simulink model "Hood_HVAC_HIL"  (R2020b)
settings: Solver=VariableStepAuto  StartTime=0.0  StopTime=inf  RelTol=1e-3
libraries: simulink x2
settings Model: Creator=99003785  LastModifiedBy=99003785

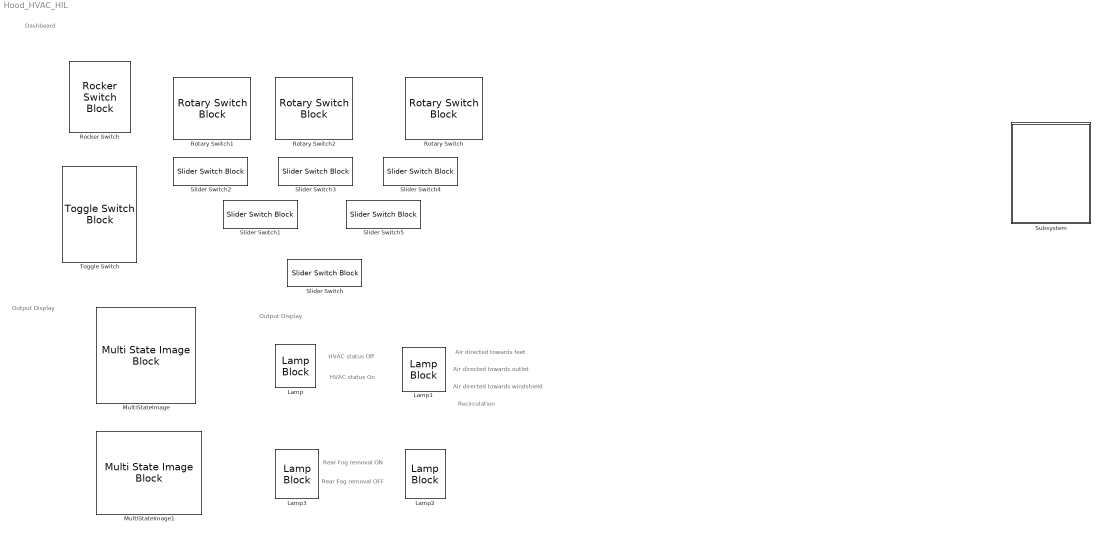
== system Hood_HVAC_HIL ==
  note: Rear Fog removal ON
  note: Air directed towards feet
  note: Air directed towards outlet
  note: HVAC status Off
  note: Output Display
  note: Recirculation
  note: Output Display
  note: Air directed towards windshield
  note: Dashboard
  note: HVAC status On
  note: Rear Fog removal OFF
  Lamp{,1..3} (4 alike) : LampBlock
  MultiStateImage : MultiStateImageBlock
  MultiStateImage1 : MultiStateImageBlock
  Rocker Switch : RockerSwitchBlock
      settings: Values={{'On', 'Off'}, [1 0]}
  Rotary Switch : RotarySwitchBlock
      settings: Values={{'Off', 'Low', 'Medium', 'High'}, [0 1 2 3]}
  Rotary Switch1 : RotarySwitchBlock
      settings: Values={{'Off', 'Low', 'Medium', 'High'}, [0 1 2 3]}
  Rotary Switch2 : RotarySwitchBlock
      settings: Values={{'Off', 'AC', 'Heater', 'Air-Vent'}, [0 1 2 3]}
  Slider Switch{,1..5} (6 alike) : SliderSwitchBlock
      settings: Values={{'Off', 'On'}, [0 1]}
  Subsystem : Subsystem
  Toggle Switch : ToggleSwitchBlock
      settings: Values={{'Off', 'On'}, [0 1]}

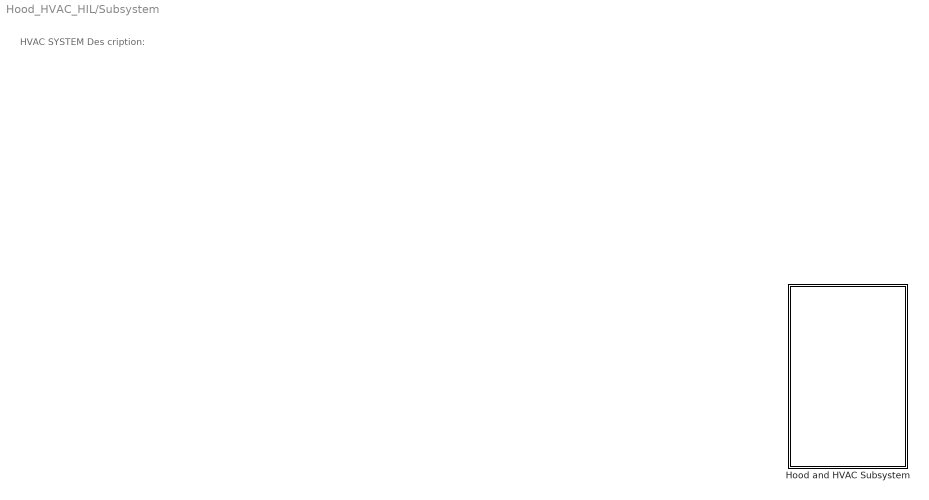
== system Hood_HVAC_HIL/Subsystem ==
  note: HVAC SYSTEM
      |
      | Des cription:
  Hood and HVAC Subsystem : Subsystem  TreatAsAtomicUnit=on

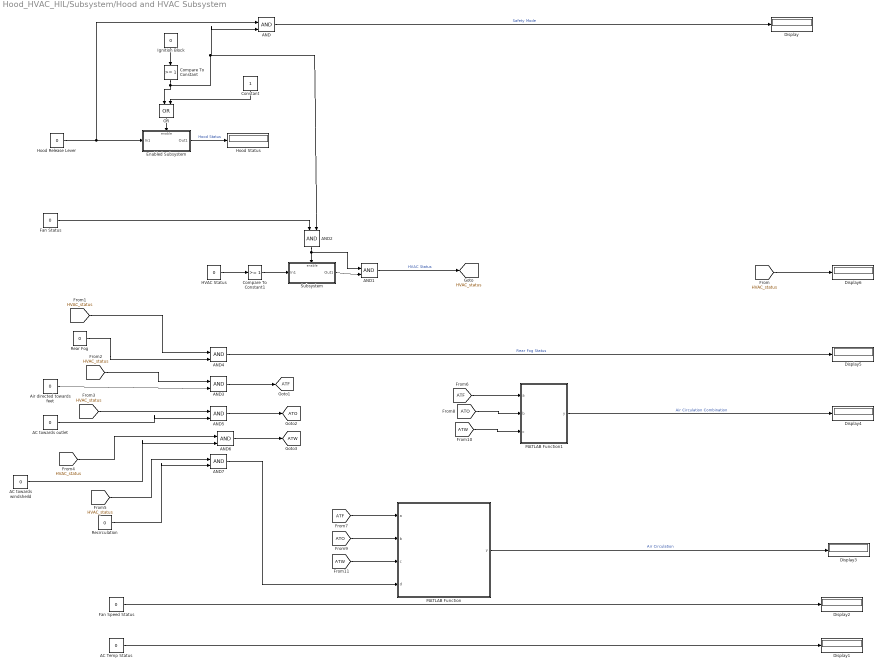
== system Hood_HVAC_HIL/Subsystem/Hood and HVAC Subsystem ==
  AC Temp Status : Constant  Value=0
  AC towards outlet : Constant  Value=0
  AC towards windsheild : Constant  Value=0
  AND{,1..7} (8 alike) : Logic  IconShape=distinctive  AllPortsSameDT=off  OutDataTypeStr=boolean
  Air directed towards feet : Constant  Value=0
  Compare To Constant : simulink/Logic and Bit Operations/Compare To Constant  relop=>=  const=1  OutDataTypeStr=boolean
  Compare To Constant1 : simulink/Logic and Bit Operations/Compare To Constant  relop=>=  const=1  OutDataTypeStr=boolean
  Constant : Constant
  Display{,1..6} (7 alike) : Display
  Enabled Subsystem : Subsystem  TreatAsAtomicUnit=on
  Fan Speed Status : Constant  Value=0
  Fan Status : Constant  Value=0
  HVAC Status : Constant  Value=0
  Hood Release Lever : Constant  Value=0
  Hood Status : Display
  Ignition Block : Constant  Value=0
  MATLAB Function : MATLAB Function  TreatAsAtomicUnit=on
  MATLAB Function1 : MATLAB Function  TreatAsAtomicUnit=on
  OR : Logic  Operator=OR  IconShape=distinctive  AllPortsSameDT=off  OutDataTypeStr=boolean
  Rear Fog : Constant  Value=0
  Recirculation : Constant  Value=0
  Subsystem : Subsystem
  tag scope: ATF=global, ATO=global, ATW=global, HVAC_status=global
  wires:
  Ignition Block/1 -> Compare To Constant/1
  AND/1 -> Display/1  "Safety Mode"
  Hood Release Lever/1 -> AND/1, Enabled Subsystem/1(In1)
  Compare To Constant/1 -> AND2/2, AND/2, OR/1
  OR/1 -> Enabled Subsystem/Enable
  Enabled Subsystem/1(Out1) -> Hood Status/1  "Hood Status"
  Constant/1 -> OR/2
  AND1/1 -> [HVAC_status]  "HVAC Status"
  Subsystem/1(Out1) -> AND1/2
  AND2/1 -> AND1/1, Subsystem/Enable
  Compare To Constant1/1 -> Subsystem/1(In1)
  HVAC Status/1 -> Compare To Constant1/1
  Recirculation/1 -> AND7/2
  AND4/1 -> Display5/1  "Rear Fog Status"
  Rear Fog/1 -> AND4/2
  AC towards outlet/1 -> AND5/2
  Air directed towards feet/1 -> AND3/2
  AC towards windsheild/1 -> AND6/2
  MATLAB Function/1(y) -> Display3/1  "Air Circulation"
  AND7/1 -> MATLAB Function/4(d)
  MATLAB Function1/1(y) -> Display4/1  "Air Circulation Combination"
  AC Temp Status/1 -> Display1/1
  Fan Speed Status/1 -> Display2/1
  Fan Status/1 -> AND2/1
  [HVAC_status] -> Display6/1
  [HVAC_status] -> AND4/1
  [HVAC_status] -> AND3/1
  [HVAC_status] -> AND5/1
  [HVAC_status] -> AND6/1
  [HVAC_status] -> AND7/1
  AND3/1 -> [ATF]
  [ATF] -> MATLAB Function1/1(a)
  [ATF] -> MATLAB Function/1(a)
  AND5/1 -> [ATO]
  [ATO] -> MATLAB Function1/2(b)
  [ATO] -> MATLAB Function/2(b)
  AND6/1 -> [ATW]
  [ATW] -> MATLAB Function1/3(c)
  [ATW] -> MATLAB Function/3(c)

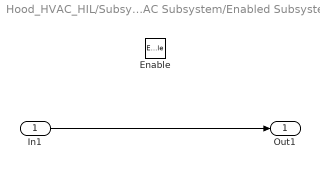
== system Hood_HVAC_HIL/Subsystem/Hood and HVAC Subsystem/Enabled Subsystem ==
  In1 : Inport
  Enable : EnablePort
  Out1 : Outport  InitialOutput=0  VectorParamsAs1DForOutWhenUnconnected=off
  wires:
  In1/1 -> Out1/1

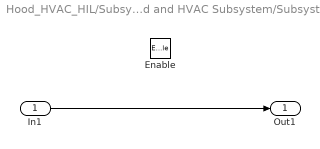
== system Hood_HVAC_HIL/Subsystem/Hood and HVAC Subsystem/Subsystem ==
  In1 : Inport
  Enable : EnablePort
  Out1 : Outport
  wires:
  In1/1 -> Out1/1

== matlab function Hood_HVAC_HIL/Subsystem/Hood and HVAC Subsystem/MATLAB Function1 ==
  data: a input; b input; c input; y output
function y = fcn(a,b,c)
    if a==1&& b==1 && c==1
        y=1;
    elseif a==1 && b==1 && c==0
        y=2;
    elseif a==1 && b==0 && c==1
        y=3;
    elseif a==0 && b==1 && c==1
        y=4;
    else
        y=0;
    end

end

== matlab function Hood_HVAC_HIL/Subsystem/Hood and HVAC Subsystem/MATLAB Function ==
  data: a input; b input; y output; c input; d input
function y = fcn(a, b, c, d)
    if a==1 && b==0 && c==0 && d==0
        y=1;
    elseif a==0 && b==1 &&c==0 && d==0
        y=2;
    elseif a==0 && b==0 &&c==1 && d==0
        y=3;
    elseif a==0 && b==0 &&c==0 && d==1
        y=4;
    else
        y=0;
    end
    

end
